simulink model "sampleModel25"  (Simulink 9.1)
settings: Solver=VariableStepAuto  StartTime=0.0  StopTime=10.0  RelTol=1e-3
undefined symbols (not defined in the file): DiscIntNeverNeededParam, Newton, Raphson
libraries: simulink x56
(part 2 of 2)

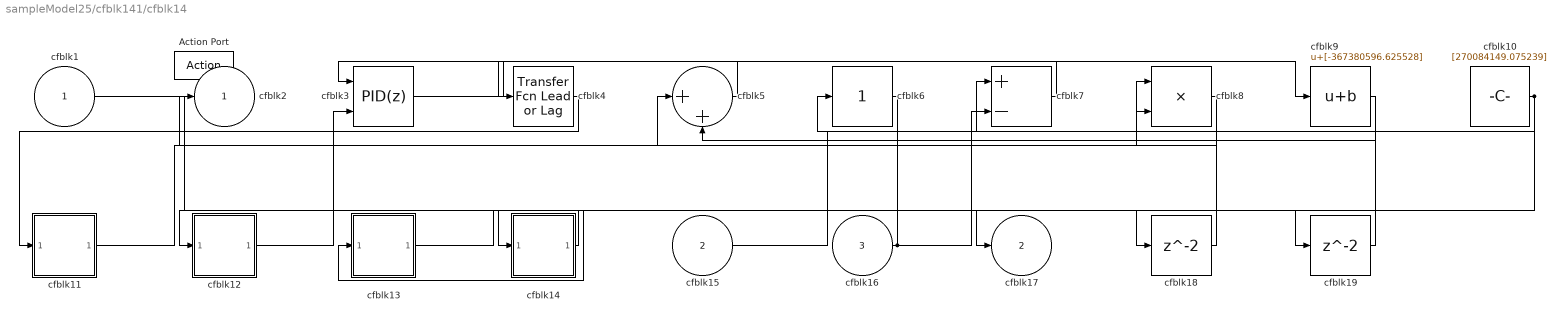
== system sampleModel25/cfblk141/cfblk14 ==
  cfblk1 : Inport
  cfblk15 : Inport  Port=2
  cfblk16 : Inport  Port=3
  Action Port : ActionPort  ActionType=then
  cfblk10 : Constant  Value=[270084149.075239]  SampleTime=1
  cfblk11 : Subsystem
  cfblk12 : Subsystem
  cfblk13 : Subsystem
  cfblk14 : Subsystem
  cfblk18 : Delay
  cfblk19 : Delay
  cfblk3 : simulink/Continuous/PID Controller (2DOF)  Controller=PID  TimeDomain=Discrete-time  SampleTime=-1  IntegratorMethod=Forward Euler  FilterMethod=Forward Euler  Form=Parallel  UseFilter=on  ControllerParametersSource=internal  P=1  I=1  D=0  N=100  b=1  c=1  InitialConditionSource=internal  InitialConditionForIntegrator=0  InitialConditionForFilter=0  ExternalReset=none  LimitOutput=off  UpperSaturationLimit=inf  LowerSaturationLimit=-inf  LinearizeAsGain=off  AntiWindupMode=none  Kb=1  TrackingMode=off  Kt=1  PParamMin=[]  PParamMax=[]  IParamMin=[]  IParamMax=[]  DParamMin=[]  DParamMax=[]  NParamMin=[]  NParamMax=[]  bParamMin=[]  bParamMax=[]  cParamMin=[]  cParamMax=[]  KbParamMin=[]  KbParamMax=[]  KtParamMin=[]  KtParamMax=[]  POutMin=[]  POutMax=[]  IOutMin=[]  IOutMax=[]  DOutMin=[]  DOutMax=[]  NOutMin=[]  NOutMax=[]  bOutMin=[]  bOutMax=[]  cOutMin=[]  cOutMax=[]  KbOutMin=[]  KbOutMax=[]  KtOutMin=[]  KtOutMax=[]  IntegratorOutMin=[]  IntegratorOutMax=[]  FilterOutMin=[]  FilterOutMax=[]  SumOutMin=[]  SumOutMax=[]  Sum1OutMin=[]  Sum1OutMax=[]  Sum2OutMin=[]  Sum2OutMax=[]  Sum3OutMin=[]  Sum3OutMax=[]  SumI1OutMin=[]  SumI1OutMax=[]  SumI2OutMin=[]  SumI2OutMax=[]  SumI3OutMin=[]  SumI3OutMax=[]  SumDOutMin=[]  SumDOutMax=[]  SaturationOutMin=[]  SaturationOutMax=[]  IntegratorContinuousStateAttributes=''  IntegratorStateMustResolveToSignalObject=off  IntegratorRTWStateStorageClass=Auto  FilterContinuousStateAttributes=''  FilterStateMustResolveToSignalObject=off  FilterRTWStateStorageClass=Auto  DifferentiatorICPrevScaledInput=0  DifferentiatorOutMin=[]  DifferentiatorOutMax=[]  FilterDiffOutCoefMin=[]  FilterDiffOutCoefMax=[]  SumDenOutMin=[]  SumDenOutMax=[]  SumNumOutMin=[]  SumNumOutMax=[]  ReciprocalOutMin=[]  ReciprocalOutMax=[]  DivideOutMin=[]  DivideOutMax=[]  TunerSelectOption=Transfer Function Based (PID Tuner App)
  cfblk4 : simulink/Discrete/Transfer Fcn Lead or Lag  PoleZ=0.95  ZeroZ=0.75  ICPrevOutput=0.0  ICPrevInput=0.0  DoSatur=off
      settings: SourceProductName=Simulink  SourceProductBaseCode=SL
  cfblk5 : Sum  Inputs=|++
  cfblk6 : simulink/Math Operations/Slider Gain  gain=1  low=0  high=2
  cfblk7 : Sum  Inputs=+-
  cfblk8 : Product  Inputs=**
  cfblk9 : Bias  Bias=[-367380596.625528]
  cfblk2 : Outport
  cfblk17 : Outport  Port=2
  wires:
  cfblk3/1 -> cfblk9/1
  cfblk4/1 -> cfblk11/1(cfblk1)
  cfblk1/1 -> cfblk14/1(cfblk1)
  cfblk5/1 -> cfblk4/1
  cfblk6/1 -> cfblk13/1(cfblk1)
  cfblk7/1 -> cfblk3/1
  cfblk14/1(cfblk2) -> cfblk12/1(cfblk1)
  cfblk12/1(cfblk2) -> cfblk3/2
  cfblk10/1 -> cfblk17/1, cfblk8/2
  cfblk9/1 -> cfblk5/2
  cfblk11/1(cfblk2) -> cfblk8/1
  cfblk15/1 -> cfblk7/1
  cfblk16/1 -> cfblk7/2, cfblk2/1
  cfblk8/1 -> cfblk18/1
  cfblk18/1 -> cfblk5/1
  cfblk13/1(cfblk2) -> cfblk19/1
  cfblk19/1 -> cfblk6/1

== system sampleModel25/cfblk141/cfblk15 ==
  cfblk1 : Inport
  cfblk12 : Inport  Port=2
  cfblk13 : Inport  Port=3
  cfblk14 : Inport  Port=4
  Action Port : ActionPort  ActionType=else
  cfblk10 : Subsystem
  cfblk11 : Subsystem
  cfblk3 : DiscreteFir
  cfblk4 : simulink/Discrete/Tapped Delay  vinit=0.0  samptime=-1  NumDelays=1  DelayOrder=Oldest  includeCurrent=off
  cfblk5 : simulink/Continuous/PID Controller (2DOF)  Controller=PID  TimeDomain=Discrete-time  SampleTime=-1  IntegratorMethod=Forward Euler  FilterMethod=Forward Euler  Form=Parallel  UseFilter=on  ControllerParametersSource=internal  P=1  I=1  D=0  N=100  b=1  c=1  InitialConditionSource=internal  InitialConditionForIntegrator=0  InitialConditionForFilter=0  ExternalReset=none  LimitOutput=off  UpperSaturationLimit=inf  LowerSaturationLimit=-inf  LinearizeAsGain=off  AntiWindupMode=none  Kb=1  TrackingMode=off  Kt=1  PParamMin=[]  PParamMax=[]  IParamMin=[]  IParamMax=[]  DParamMin=[]  DParamMax=[]  NParamMin=[]  NParamMax=[]  bParamMin=[]  bParamMax=[]  cParamMin=[]  cParamMax=[]  KbParamMin=[]  KbParamMax=[]  KtParamMin=[]  KtParamMax=[]  POutMin=[]  POutMax=[]  IOutMin=[]  IOutMax=[]  DOutMin=[]  DOutMax=[]  NOutMin=[]  NOutMax=[]  bOutMin=[]  bOutMax=[]  cOutMin=[]  cOutMax=[]  KbOutMin=[]  KbOutMax=[]  KtOutMin=[]  KtOutMax=[]  IntegratorOutMin=[]  IntegratorOutMax=[]  FilterOutMin=[]  FilterOutMax=[]  SumOutMin=[]  SumOutMax=[]  Sum1OutMin=[]  Sum1OutMax=[]  Sum2OutMin=[]  Sum2OutMax=[]  Sum3OutMin=[]  Sum3OutMax=[]  SumI1OutMin=[]  SumI1OutMax=[]  SumI2OutMin=[]  SumI2OutMax=[]  SumI3OutMin=[]  SumI3OutMax=[]  SumDOutMin=[]  SumDOutMax=[]  SaturationOutMin=[]  SaturationOutMax=[]  IntegratorContinuousStateAttributes=''  IntegratorStateMustResolveToSignalObject=off  IntegratorRTWStateStorageClass=Auto  FilterContinuousStateAttributes=''  FilterStateMustResolveToSignalObject=off  FilterRTWStateStorageClass=Auto  DifferentiatorICPrevScaledInput=0  DifferentiatorOutMin=[]  DifferentiatorOutMax=[]  FilterDiffOutCoefMin=[]  FilterDiffOutCoefMax=[]  SumDenOutMin=[]  SumDenOutMax=[]  SumNumOutMin=[]  SumNumOutMax=[]  ReciprocalOutMin=[]  ReciprocalOutMax=[]  DivideOutMin=[]  DivideOutMax=[]  TunerSelectOption=Transfer Function Based (PID Tuner App)
  cfblk6 : Abs
  cfblk7 : ComplexToMagnitudeAngle
  cfblk8 : Constant  Value=[-68296175.409686]  SampleTime=1
  cfblk9 : Subsystem
  cfblk2 : Outport
  cfblk15 : Outport  Port=2
  wires:
  cfblk6/1 -> cfblk5/1
  cfblk9/1(cfblk2) -> cfblk11/1(cfblk1)
  cfblk10/1(cfblk2) -> cfblk5/2
  cfblk8/1 -> cfblk4/1
  cfblk13/1 -> cfblk7/1
  cfblk5/1 -> cfblk9/1(cfblk1)
  cfblk4/1 -> cfblk3/1
  cfblk14/1 -> cfblk15/1
  cfblk12/1 -> cfblk2/1
  cfblk1/1 -> cfblk6/1
  cfblk3/1 -> cfblk10/1(cfblk1)

== system sampleModel25/cfblk141/cfblk6 ==
  cfblk1 : Inport
  cfblk2 : Outport
  wires:
  cfblk1/1 -> cfblk2/1

== system sampleModel25/cfblk141/cfblk7 ==
  cfblk1 : Inport
  cfblk2 : Outport
  wires:
  cfblk1/1 -> cfblk2/1

== system sampleModel25/cfblk142/cfblk8 ==
  cfblk1 : Inport
  cfblk2 : Outport
  wires:
  cfblk1/1 -> cfblk2/1

== system sampleModel25/cfblk143/cfblk10 ==
  cfblk1 : Inport
  cfblk2 : Outport
  wires:
  cfblk1/1 -> cfblk2/1

== system sampleModel25/cfblk143/cfblk11 ==
  cfblk1 : Inport
  cfblk2 : Outport
  wires:
  cfblk1/1 -> cfblk2/1

== system sampleModel25/cfblk143/cfblk12 ==
  cfblk1 : Inport
  cfblk2 : Outport
  wires:
  cfblk1/1 -> cfblk2/1

== system sampleModel25/cfblk143/cfblk9 ==
  cfblk1 : Inport
  cfblk2 : Outport
  wires:
  cfblk1/1 -> cfblk2/1

== system sampleModel25/cfblk144/cfblk11 ==
  cfblk1 : Inport
  cfblk2 : Outport
  wires:
  cfblk1/1 -> cfblk2/1

== system sampleModel25/cfblk144/cfblk12 ==
  cfblk1 : Inport
  cfblk2 : Outport
  wires:
  cfblk1/1 -> cfblk2/1

== system sampleModel25/cfblk144/cfblk13 ==
  cfblk1 : Inport
  cfblk2 : Outport
  wires:
  cfblk1/1 -> cfblk2/1

== system sampleModel25/cfblk144/cfblk14 ==
  cfblk1 : Inport
  cfblk2 : Outport
  wires:
  cfblk1/1 -> cfblk2/1

== system sampleModel25/cfblk144/cfblk18 ==
  cfblk1 : Inport
  Action Port : ActionPort  ActionType=then
  cfblk3 : MinMax  Function=max  Inputs=2
  cfblk4 : Subsystem
  cfblk5 : Subsystem
  cfblk6 : Subsystem
  cfblk7 : Subsystem
  cfblk8 : Subsystem
  cfblk9 : Delay
  cfblk2 : Outport
  wires:
  cfblk8/1(cfblk2) -> cfblk4/1(cfblk1), cfblk7/1(cfblk1)
  cfblk6/1(cfblk2) -> cfblk8/1(cfblk1)
  cfblk1/1 -> cfblk3/1
  cfblk4/1(cfblk2) -> cfblk2/1
  cfblk3/1 -> cfblk5/1(cfblk1)
  cfblk5/1(cfblk2) -> cfblk6/1(cfblk1)
  cfblk7/1(cfblk2) -> cfblk9/1
  cfblk9/1 -> cfblk3/2

== system sampleModel25/cfblk144/cfblk19 ==
  cfblk1 : Inport
  cfblk7 : Inport  Port=2
  cfblk8 : Inport  Port=3
  Action Port : ActionPort  ActionType=else
  cfblk3 : simulink/Discrete/Transfer Fcn Lead or Lag  PoleZ=0.95  ZeroZ=0.75  ICPrevOutput=0.0  ICPrevInput=0.0  DoSatur=off
      settings: SourceProductName=Simulink  SourceProductBaseCode=SL
  cfblk4 : ComplexToRealImag
  cfblk5 : DotProduct  InputSameDT=on  OutDataTypeStr=Inherit: Inherit via internal rule
  cfblk6 : Subsystem
  cfblk2 : Outport
  wires:
  cfblk1/1 -> cfblk4/1
  cfblk3/1 -> cfblk2/1
  cfblk8/1 -> cfblk3/1
  cfblk7/1 -> cfblk5/1
  cfblk4/1 -> cfblk5/2
  cfblk4/2 -> cfblk6/1(cfblk1)

== system sampleModel25/cfblk145/cfblk10 ==
  cfblk1 : Inport
  cfblk2 : Outport
  wires:
  cfblk1/1 -> cfblk2/1

== system sampleModel25/cfblk145/cfblk7 ==
  cfblk1 : Inport
  cfblk2 : Outport
  wires:
  cfblk1/1 -> cfblk2/1

== system sampleModel25/cfblk145/cfblk8 ==
  cfblk1 : Inport
  cfblk2 : Outport
  wires:
  cfblk1/1 -> cfblk2/1

== system sampleModel25/cfblk145/cfblk9 ==
  cfblk1 : Inport
  cfblk2 : Outport
  wires:
  cfblk1/1 -> cfblk2/1

== system sampleModel25/cfblk146/cfblk9 ==
  cfblk1 : Inport
  cfblk2 : Outport
  wires:
  cfblk1/1 -> cfblk2/1

== system sampleModel25/cfblk147/cfblk10 ==
  cfblk1 : Inport
  cfblk2 : Outport
  wires:
  cfblk1/1 -> cfblk2/1

== system sampleModel25/cfblk147/cfblk18 ==
  cfblk1 : Inport
  cfblk6 : Inport  Port=2
  cfblk7 : Inport  Port=3
  cfblk8 : Inport  Port=4
  cfblk9 : Inport  Port=5
  Action Port : ActionPort  ActionType=then
  cfblk3 : Product  Inputs=**
  cfblk4 : Subsystem
  cfblk5 : Subsystem
  cfblk2 : Outport
  cfblk10 : Outport  Port=2
  cfblk11 : Outport  Port=3
  wires:
  cfblk7/1 -> cfblk3/1
  cfblk4/1(cfblk2) -> cfblk2/1
  cfblk3/1 -> cfblk10/1
  cfblk8/1 -> cfblk3/2
  cfblk9/1 -> cfblk5/1(cfblk1)
  cfblk5/1(cfblk2) -> cfblk4/1(cfblk1)
  cfblk6/1 -> cfblk11/1

== system sampleModel25/cfblk147/cfblk19 ==
  cfblk1 : Inport
  Action Port : ActionPort  ActionType=else
  cfblk10 : Subsystem
  cfblk11 : Subsystem
  cfblk12 : Subsystem
  cfblk3 : DiscreteFilter
  cfblk4 : DiscreteTransferFcn
  cfblk5 : Sum  Inputs=+
  cfblk6 : Sum  Inputs=|++
  cfblk7 : Subsystem
  cfblk8 : Subsystem
  cfblk9 : Subsystem
  cfblk2 : Outport
  cfblk13 : Outport  Port=2
  wires:
  cfblk8/1(cfblk2) -> cfblk10/1(cfblk1)
  cfblk1/1 -> cfblk3/1
  cfblk10/1(cfblk2) -> cfblk13/1
  cfblk5/1 -> cfblk8/1(cfblk1)
  cfblk6/1 -> cfblk7/1(cfblk1)
  cfblk7/1(cfblk2) -> cfblk9/1(cfblk1)
  cfblk3/1 -> cfblk4/1
  cfblk9/1(cfblk2) -> cfblk11/1(cfblk1)
  cfblk4/1 -> cfblk6/1, cfblk6/2
  cfblk11/1(cfblk2) -> cfblk5/1, cfblk12/1(cfblk1)
  cfblk12/1(cfblk2) -> cfblk2/1

== system sampleModel25/cfblk148/cfblk7 ==
  cfblk1 : Inport
  cfblk2 : Outport
  wires:
  cfblk1/1 -> cfblk2/1

== system sampleModel25/cfblk149/cfblk10 ==
  cfblk1 : Inport
  cfblk2 : Outport
  wires:
  cfblk1/1 -> cfblk2/1

== system sampleModel25/cfblk149/cfblk11 ==
  cfblk1 : Inport
  cfblk2 : Outport
  wires:
  cfblk1/1 -> cfblk2/1

== system sampleModel25/cfblk149/cfblk8 ==
  cfblk1 : Inport
  cfblk2 : Outport
  wires:
  cfblk1/1 -> cfblk2/1

== system sampleModel25/cfblk149/cfblk9 ==
  cfblk1 : Inport
  cfblk2 : Outport
  wires:
  cfblk1/1 -> cfblk2/1

== system sampleModel25/cfblk140/cfblk13/cfblk10 ==
  cfblk1 : Inport
  cfblk2 : Outport
  wires:
  cfblk1/1 -> cfblk2/1

== system sampleModel25/cfblk140/cfblk13/cfblk11 ==
  cfblk1 : Inport
  cfblk2 : Outport
  wires:
  cfblk1/1 -> cfblk2/1

== system sampleModel25/cfblk140/cfblk13/cfblk12 ==
  cfblk1 : Inport
  cfblk2 : Outport
  wires:
  cfblk1/1 -> cfblk2/1

== system sampleModel25/cfblk140/cfblk13/cfblk13 ==
  cfblk1 : Inport
  cfblk2 : Outport
  wires:
  cfblk1/1 -> cfblk2/1

== system sampleModel25/cfblk140/cfblk13/cfblk9 ==
  cfblk1 : Inport
  cfblk2 : Outport
  wires:
  cfblk1/1 -> cfblk2/1

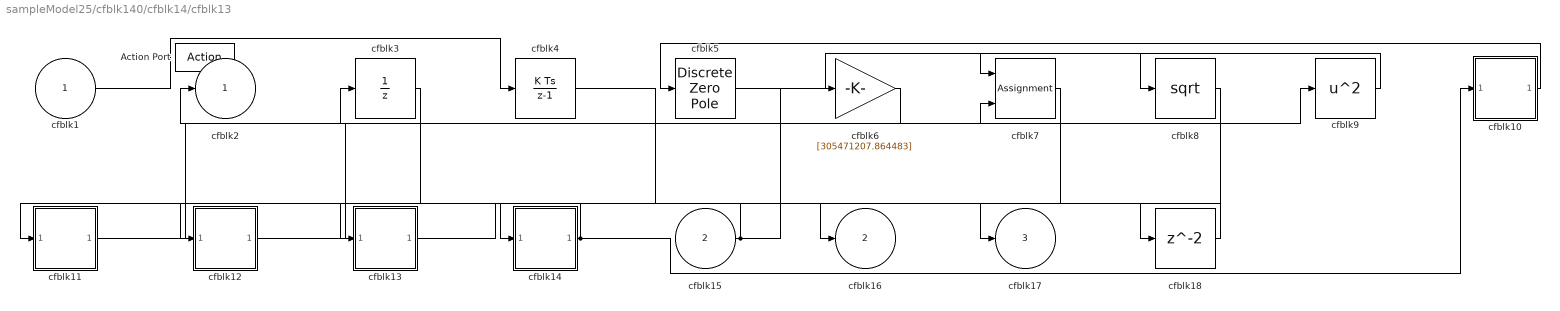
== system sampleModel25/cfblk140/cfblk14/cfblk13 ==
  cfblk1 : Inport
  cfblk15 : Inport  Port=2
  Action Port : ActionPort  ActionType=then
  cfblk10 : Subsystem
  cfblk11 : Subsystem
  cfblk12 : Subsystem
  cfblk13 : Subsystem
  cfblk14 : Subsystem
  cfblk18 : Delay
  cfblk3 : UnitDelay  SampleTime=-1
  cfblk4 : DiscreteIntegrator  SampleTime=-1  ICPrevOutput=DiscIntNeverNeededParam  ICPrevScaledInput=DiscIntNeverNeededParam
  cfblk5 : DiscreteZeroPole  Poles=[0 0.5]  Gain=1  SampleTime=-1
  cfblk6 : Gain  Gain=[305471207.864483]
  cfblk7 : Assignment  DiagnosticForDimensions=Warning  IndexOptions=Index vector (dialog)  Indices=1  OutputSizes=1
  cfblk8 : Sqrt  SaturateOnIntegerOverflow=on
  cfblk9 : Math  Operator=square  SaturateOnIntegerOverflow=on
  cfblk2 : Outport
  cfblk16 : Outport  Port=2
  cfblk17 : Outport  Port=3
  wires:
  cfblk5/1 -> cfblk8/1
  cfblk12/1(cfblk2) -> cfblk9/1
  cfblk1/1 -> cfblk4/1
  cfblk6/1 -> cfblk2/1
  cfblk15/1 -> cfblk14/1(cfblk1), cfblk6/1
  cfblk9/1 -> cfblk7/1
  cfblk14/1(cfblk2) -> cfblk10/1(cfblk1), cfblk11/1(cfblk1)
  cfblk7/1 -> cfblk13/1(cfblk1)
  cfblk8/1 -> cfblk16/1
  cfblk11/1(cfblk2) -> cfblk3/1
  cfblk10/1(cfblk2) -> cfblk5/1
  cfblk4/1 -> cfblk17/1
  cfblk3/1 -> cfblk12/1(cfblk1)
  cfblk13/1(cfblk2) -> cfblk18/1
  cfblk18/1 -> cfblk7/2

== system sampleModel25/cfblk140/cfblk14/cfblk14 ==
  cfblk1 : Inport
  cfblk11 : Inport  Port=2
  Action Port : ActionPort  ActionType=else
  cfblk10 : Subsystem
  cfblk3 : simulink/Discrete/Transfer Fcn Lead or Lag  PoleZ=0.95  ZeroZ=0.75  ICPrevOutput=0.0  ICPrevInput=0.0  DoSatur=off
      settings: SourceProductName=Simulink  SourceProductBaseCode=SL
  cfblk4 : Sin  TimeSource=Use external signal  SampleTime=0
  cfblk5 : Constant  Value=[13372239.767599]  SampleTime=1
  cfblk6 : Constant  Value=[-888197703.177036]  SampleTime=1
  cfblk7 : Subsystem
  cfblk8 : Subsystem
  cfblk9 : Subsystem
  cfblk2 : Outport
  cfblk12 : Outport  Port=2
  wires:
  cfblk1/1 -> cfblk4/1
  cfblk8/1(cfblk2) -> cfblk12/1
  cfblk4/1 -> cfblk8/1(cfblk1)
  cfblk9/1(cfblk2) -> cfblk7/1(cfblk1)
  cfblk5/1 -> cfblk3/1
  cfblk6/1 -> cfblk9/1(cfblk1)
  cfblk3/1 -> cfblk2/1
  cfblk7/1(cfblk2) -> cfblk10/1(cfblk1)

== system sampleModel25/cfblk140/cfblk14/cfblk6 ==
  cfblk1 : Inport
  cfblk2 : Outport
  wires:
  cfblk1/1 -> cfblk2/1

== system sampleModel25/cfblk140/cfblk14/cfblk7 ==
  cfblk1 : Inport
  cfblk2 : Outport
  wires:
  cfblk1/1 -> cfblk2/1

== system sampleModel25/cfblk140/cfblk14/cfblk8 ==
  cfblk1 : Inport
  cfblk2 : Outport
  wires:
  cfblk1/1 -> cfblk2/1

== system sampleModel25/cfblk140/cfblk15/cfblk9 ==
  cfblk1 : Inport
  cfblk2 : Outport
  wires:
  cfblk1/1 -> cfblk2/1

== system sampleModel25/cfblk140/cfblk16/cfblk6 ==
  cfblk1 : Inport
  cfblk2 : Outport
  wires:
  cfblk1/1 -> cfblk2/1

== system sampleModel25/cfblk140/cfblk16/cfblk7 ==
  cfblk1 : Inport
  cfblk2 : Outport
  wires:
  cfblk1/1 -> cfblk2/1

== system sampleModel25/cfblk141/cfblk12/cfblk10 ==
  cfblk1 : Inport
  cfblk2 : Outport
  wires:
  cfblk1/1 -> cfblk2/1

== system sampleModel25/cfblk141/cfblk12/cfblk11 ==
  cfblk1 : Inport
  cfblk2 : Outport
  wires:
  cfblk1/1 -> cfblk2/1

== system sampleModel25/cfblk141/cfblk12/cfblk16 ==
  cfblk1 : Inport
  Action Port : ActionPort  ActionType=then
  cfblk3 : Sqrt  SaturateOnIntegerOverflow=on
  cfblk4 : simulink/Math Operations/MinMax Running Resettable  Function=min  vinit=0.0
  cfblk5 : Constant  Value=[222304569.355251]  SampleTime=1
  cfblk6 : Constant  Value=[-506290689.066987]  SampleTime=1
  cfblk7 : Subsystem
  cfblk8 : Subsystem
  cfblk2 : Outport
  cfblk9 : Outport  Port=2
  wires:
  cfblk6/1 -> cfblk7/1(cfblk1)
  cfblk8/1(cfblk2) -> cfblk9/1
  cfblk5/1 -> cfblk2/1
  cfblk7/1(cfblk2) -> cfblk3/1
  cfblk3/1 -> cfblk4/1
  cfblk4/1 -> cfblk8/1(cfblk1)
  cfblk1/1 -> cfblk4/2

== system sampleModel25/cfblk141/cfblk12/cfblk17 ==
  cfblk1 : Inport
  cfblk13 : Inport  Port=2
  cfblk14 : Inport  Port=3
  cfblk15 : Inport  Port=4
  Action Port : ActionPort  ActionType=else
  cfblk10 : Subsystem
  cfblk11 : Subsystem
  cfblk12 : Subsystem
  cfblk3 : simulink/Discrete/Difference  ICPrevInput=0.0  OutMin=[]  OutMax=[]  OutDataTypeStr=Inherit: Inherit via back propagation  OutDataType=fixdt(1, 16)  OutScaling=2^-10  DoSatur=off
  cfblk4 : simulink/Discrete/Difference  ICPrevInput=0.0  OutMin=[]  OutMax=[]  OutDataTypeStr=Inherit: Inherit via back propagation  OutDataType=fixdt(1, 16)  OutScaling=2^-10  DoSatur=off
  cfblk5 : simulink/Discrete/Transfer Fcn First Order  PoleZ=0.95  ICPrevOutput=0.0  DoSatur=off
      settings: SourceProductName=Simulink
  cfblk6 : Bias  Bias=[920258495.168729]
  cfblk7 : Abs
  cfblk8 : Subsystem
  cfblk9 : Subsystem
  cfblk2 : Outport
  wires:
  cfblk6/1 -> cfblk7/1
  cfblk12/1(cfblk2) -> cfblk2/1
  cfblk1/1 -> cfblk12/1(cfblk1)
  cfblk5/1 -> cfblk4/1
  cfblk8/1(cfblk2) -> cfblk5/1
  cfblk10/1(cfblk2) -> cfblk11/1(cfblk1)
  cfblk11/1(cfblk2) -> cfblk8/1(cfblk1)
  cfblk3/1 -> cfblk6/1
  cfblk9/1(cfblk2) -> cfblk3/1
  cfblk13/1 -> cfblk10/1(cfblk1)
  cfblk15/1 -> cfblk9/1(cfblk1)

== system sampleModel25/cfblk141/cfblk12/cfblk9 ==
  cfblk1 : Inport
  cfblk2 : Outport
  wires:
  cfblk1/1 -> cfblk2/1

== system sampleModel25/cfblk141/cfblk13/cfblk10 ==
  cfblk1 : Inport
  cfblk2 : Outport
  wires:
  cfblk1/1 -> cfblk2/1

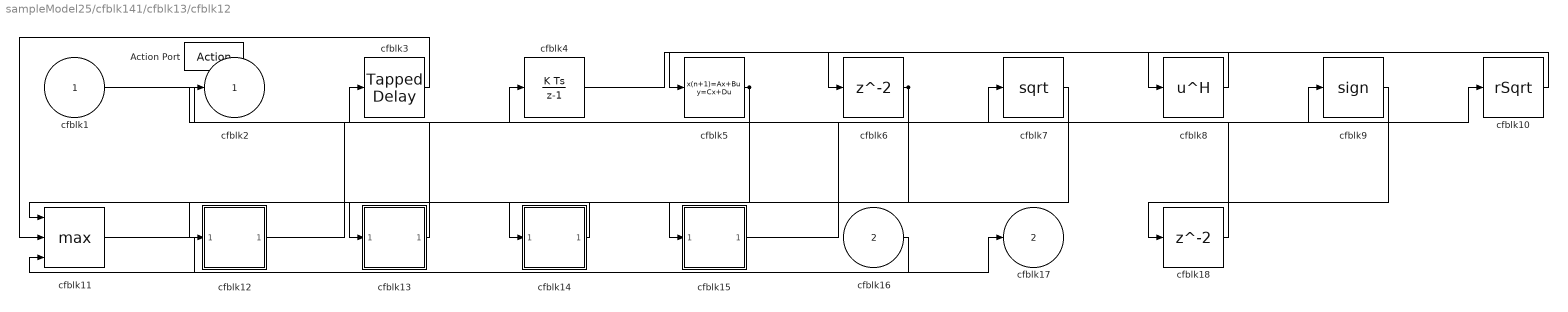
== system sampleModel25/cfblk141/cfblk13/cfblk12 ==
  cfblk1 : Inport
  cfblk16 : Inport  Port=2
  Action Port : ActionPort  ActionType=then
  cfblk10 : Sqrt  Operator=rSqrt  AlgorithmType=Newton-Raphson  SaturateOnIntegerOverflow=on
  cfblk11 : MinMax  Function=max  Inputs=3
  cfblk12 : Subsystem
  cfblk13 : Subsystem
  cfblk14 : Subsystem
  cfblk15 : Subsystem
  cfblk18 : Delay
  cfblk3 : simulink/Discrete/Tapped Delay  vinit=0.0  samptime=-1  NumDelays=1  DelayOrder=Oldest  includeCurrent=off
  cfblk4 : DiscreteIntegrator  SampleTime=-1  ICPrevOutput=DiscIntNeverNeededParam  ICPrevScaledInput=DiscIntNeverNeededParam
  cfblk5 : DiscreteStateSpace  SampleTime=-1
  cfblk6 : Delay
  cfblk7 : Sqrt  SaturateOnIntegerOverflow=on
  cfblk8 : Math  Operator=hermitian  SaturateOnIntegerOverflow=on
  cfblk9 : Signum
  cfblk2 : Outport
  cfblk17 : Outport  Port=2
  wires:
  cfblk6/1 -> cfblk13/1(cfblk1), cfblk15/1(cfblk1)
  cfblk10/1 -> cfblk5/1
  cfblk11/1 -> cfblk17/1
  cfblk15/1(cfblk2) -> cfblk10/1
  cfblk4/1 -> cfblk8/1
  cfblk14/1(cfblk2) -> cfblk12/1(cfblk1)
  cfblk12/1(cfblk2) -> cfblk9/1
  cfblk1/1 -> cfblk7/1
  cfblk8/1 -> cfblk6/1
  cfblk7/1 -> cfblk11/1
  cfblk13/1(cfblk2) -> cfblk3/1
  cfblk3/1 -> cfblk11/2
  cfblk5/1 -> cfblk2/1, cfblk14/1(cfblk1)
  cfblk16/1 -> cfblk11/3
  cfblk9/1 -> cfblk18/1
  cfblk18/1 -> cfblk4/1

== system sampleModel25/cfblk141/cfblk13/cfblk13 ==
  cfblk1 : Inport
  cfblk8 : Inport  Port=2
  cfblk9 : Inport  Port=3
  cfblk10 : Inport  Port=4
  cfblk11 : Inport  Port=5
  Action Port : ActionPort  ActionType=else
  cfblk3 : simulink/Discrete/Difference  ICPrevInput=0.0  OutMin=[]  OutMax=[]  OutDataTypeStr=Inherit: Inherit via back propagation  OutDataType=fixdt(1, 16)  OutScaling=2^-10  DoSatur=off
  cfblk4 : simulink/Continuous/PID Controller  Controller=PID  TimeDomain=Discrete-time  SampleTime=-1  IntegratorMethod=Forward Euler  FilterMethod=Forward Euler  Form=Parallel  UseFilter=on  ControllerParametersSource=internal  P=1  I=1  D=0  N=100  InitialConditionSource=internal  InitialConditionForIntegrator=0  InitialConditionForFilter=0  ExternalReset=none  LimitOutput=off  UpperSaturationLimit=inf  LowerSaturationLimit=-inf  LinearizeAsGain=off  AntiWindupMode=none  Kb=1  TrackingMode=off  Kt=1  PParamMin=[]  PParamMax=[]  IParamMin=[]  IParamMax=[]  DParamMin=[]  DParamMax=[]  NParamMin=[]  NParamMax=[]  KbParamMin=[]  KbParamMax=[]  KtParamMin=[]  KtParamMax=[]  POutMin=[]  POutMax=[]  IOutMin=[]  IOutMax=[]  DOutMin=[]  DOutMax=[]  NOutMin=[]  NOutMax=[]  KbOutMin=[]  KbOutMax=[]  KtOutMin=[]  KtOutMax=[]  IntegratorOutMin=[]  IntegratorOutMax=[]  FilterOutMin=[]  FilterOutMax=[]  SumOutMin=[]  SumOutMax=[]  SumI1OutMin=[]  SumI1OutMax=[]  SumI2OutMin=[]  SumI2OutMax=[]  SumI3OutMin=[]  SumI3OutMax=[]  SumDOutMin=[]  SumDOutMax=[]  SaturationOutMin=[]  SaturationOutMax=[]  IntegratorContinuousStateAttributes=''  IntegratorStateMustResolveToSignalObject=off  IntegratorRTWStateStorageClass=Auto  FilterContinuousStateAttributes=''  FilterStateMustResolveToSignalObject=off  FilterRTWStateStorageClass=Auto  DifferentiatorICPrevScaledInput=0  DifferentiatorOutMin=[]  DifferentiatorOutMax=[]  FilterDiffOutCoefMin=[]  FilterDiffOutCoefMax=[]  SumDenOutMin=[]  SumDenOutMax=[]  SumNumOutMin=[]  SumNumOutMax=[]  ReciprocalOutMin=[]  ReciprocalOutMax=[]  DivideOutMin=[]  DivideOutMax=[]  TunerSelectOption=Transfer Function Based (PID Tuner App)
  cfblk5 : Product  Inputs=**
  cfblk6 : Constant  Value=[-41324313.478639]  SampleTime=1
  cfblk7 : Subsystem
  cfblk2 : Outport
  cfblk12 : Outport  Port=2
  wires:
  cfblk6/1 -> cfblk5/1
  cfblk7/1(cfblk2) -> cfblk2/1
  cfblk5/1 -> cfblk7/1(cfblk1)
  cfblk11/1 -> cfblk5/2
  cfblk1/1 -> cfblk3/1
  cfblk9/1 -> cfblk12/1
  cfblk10/1 -> cfblk4/1

== system sampleModel25/cfblk141/cfblk13/cfblk7 ==
  cfblk1 : Inport
  cfblk2 : Outport
  wires:
  cfblk1/1 -> cfblk2/1

== system sampleModel25/cfblk141/cfblk13/cfblk8 ==
  cfblk1 : Inport
  cfblk2 : Outport
  wires:
  cfblk1/1 -> cfblk2/1

== system sampleModel25/cfblk141/cfblk13/cfblk9 ==
  cfblk1 : Inport
  cfblk2 : Outport
  wires:
  cfblk1/1 -> cfblk2/1

== system sampleModel25/cfblk141/cfblk14/cfblk11 ==
  cfblk1 : Inport
  cfblk2 : Outport
  wires:
  cfblk1/1 -> cfblk2/1

== system sampleModel25/cfblk141/cfblk14/cfblk12 ==
  cfblk1 : Inport
  cfblk2 : Outport
  wires:
  cfblk1/1 -> cfblk2/1

== system sampleModel25/cfblk141/cfblk14/cfblk13 ==
  cfblk1 : Inport
  cfblk2 : Outport
  wires:
  cfblk1/1 -> cfblk2/1

== system sampleModel25/cfblk141/cfblk14/cfblk14 ==
  cfblk1 : Inport
  cfblk2 : Outport
  wires:
  cfblk1/1 -> cfblk2/1

== system sampleModel25/cfblk141/cfblk15/cfblk10 ==
  cfblk1 : Inport
  cfblk2 : Outport
  wires:
  cfblk1/1 -> cfblk2/1

== system sampleModel25/cfblk141/cfblk15/cfblk11 ==
  cfblk1 : Inport
  cfblk2 : Outport
  wires:
  cfblk1/1 -> cfblk2/1

== system sampleModel25/cfblk141/cfblk15/cfblk9 ==
  cfblk1 : Inport
  cfblk2 : Outport
  wires:
  cfblk1/1 -> cfblk2/1

== system sampleModel25/cfblk144/cfblk18/cfblk4 ==
  cfblk1 : Inport
  cfblk2 : Outport
  wires:
  cfblk1/1 -> cfblk2/1

== system sampleModel25/cfblk144/cfblk18/cfblk5 ==
  cfblk1 : Inport
  cfblk2 : Outport
  wires:
  cfblk1/1 -> cfblk2/1

== system sampleModel25/cfblk144/cfblk18/cfblk6 ==
  cfblk1 : Inport
  cfblk2 : Outport
  wires:
  cfblk1/1 -> cfblk2/1

== system sampleModel25/cfblk144/cfblk18/cfblk7 ==
  cfblk1 : Inport
  cfblk2 : Outport
  wires:
  cfblk1/1 -> cfblk2/1

== system sampleModel25/cfblk144/cfblk18/cfblk8 ==
  cfblk1 : Inport
  cfblk2 : Outport
  wires:
  cfblk1/1 -> cfblk2/1

== system sampleModel25/cfblk144/cfblk19/cfblk6 ==
  cfblk1 : Inport
  cfblk2 : Outport
  wires:
  cfblk1/1 -> cfblk2/1

== system sampleModel25/cfblk147/cfblk18/cfblk4 ==
  cfblk1 : Inport
  cfblk2 : Outport
  wires:
  cfblk1/1 -> cfblk2/1

== system sampleModel25/cfblk147/cfblk18/cfblk5 ==
  cfblk1 : Inport
  cfblk2 : Outport
  wires:
  cfblk1/1 -> cfblk2/1

== system sampleModel25/cfblk147/cfblk19/cfblk10 ==
  cfblk1 : Inport
  cfblk2 : Outport
  wires:
  cfblk1/1 -> cfblk2/1

== system sampleModel25/cfblk147/cfblk19/cfblk11 ==
  cfblk1 : Inport
  cfblk2 : Outport
  wires:
  cfblk1/1 -> cfblk2/1

== system sampleModel25/cfblk147/cfblk19/cfblk12 ==
  cfblk1 : Inport
  cfblk2 : Outport
  wires:
  cfblk1/1 -> cfblk2/1

== system sampleModel25/cfblk147/cfblk19/cfblk7 ==
  cfblk1 : Inport
  cfblk2 : Outport
  wires:
  cfblk1/1 -> cfblk2/1

== system sampleModel25/cfblk147/cfblk19/cfblk8 ==
  cfblk1 : Inport
  cfblk2 : Outport
  wires:
  cfblk1/1 -> cfblk2/1

== system sampleModel25/cfblk147/cfblk19/cfblk9 ==
  cfblk1 : Inport
  cfblk2 : Outport
  wires:
  cfblk1/1 -> cfblk2/1

== system sampleModel25/cfblk140/cfblk14/cfblk13/cfblk10 ==
  cfblk1 : Inport
  cfblk2 : Outport
  wires:
  cfblk1/1 -> cfblk2/1

== system sampleModel25/cfblk140/cfblk14/cfblk13/cfblk11 ==
  cfblk1 : Inport
  cfblk2 : Outport
  wires:
  cfblk1/1 -> cfblk2/1

== system sampleModel25/cfblk140/cfblk14/cfblk13/cfblk12 ==
  cfblk1 : Inport
  cfblk2 : Outport
  wires:
  cfblk1/1 -> cfblk2/1

== system sampleModel25/cfblk140/cfblk14/cfblk13/cfblk13 ==
  cfblk1 : Inport
  cfblk2 : Outport
  wires:
  cfblk1/1 -> cfblk2/1

== system sampleModel25/cfblk140/cfblk14/cfblk13/cfblk14 ==
  cfblk1 : Inport
  cfblk2 : Outport
  wires:
  cfblk1/1 -> cfblk2/1

== system sampleModel25/cfblk140/cfblk14/cfblk14/cfblk10 ==
  cfblk1 : Inport
  cfblk2 : Outport
  wires:
  cfblk1/1 -> cfblk2/1

== system sampleModel25/cfblk140/cfblk14/cfblk14/cfblk7 ==
  cfblk1 : Inport
  cfblk2 : Outport
  wires:
  cfblk1/1 -> cfblk2/1

== system sampleModel25/cfblk140/cfblk14/cfblk14/cfblk8 ==
  cfblk1 : Inport
  cfblk2 : Outport
  wires:
  cfblk1/1 -> cfblk2/1

== system sampleModel25/cfblk140/cfblk14/cfblk14/cfblk9 ==
  cfblk1 : Inport
  cfblk2 : Outport
  wires:
  cfblk1/1 -> cfblk2/1

== system sampleModel25/cfblk141/cfblk12/cfblk16/cfblk7 ==
  cfblk1 : Inport
  cfblk2 : Outport
  wires:
  cfblk1/1 -> cfblk2/1

== system sampleModel25/cfblk141/cfblk12/cfblk16/cfblk8 ==
  cfblk1 : Inport
  cfblk2 : Outport
  wires:
  cfblk1/1 -> cfblk2/1

== system sampleModel25/cfblk141/cfblk12/cfblk17/cfblk10 ==
  cfblk1 : Inport
  cfblk2 : Outport
  wires:
  cfblk1/1 -> cfblk2/1

== system sampleModel25/cfblk141/cfblk12/cfblk17/cfblk11 ==
  cfblk1 : Inport
  cfblk2 : Outport
  wires:
  cfblk1/1 -> cfblk2/1

== system sampleModel25/cfblk141/cfblk12/cfblk17/cfblk12 ==
  cfblk1 : Inport
  cfblk2 : Outport
  wires:
  cfblk1/1 -> cfblk2/1

== system sampleModel25/cfblk141/cfblk12/cfblk17/cfblk8 ==
  cfblk1 : Inport
  cfblk2 : Outport
  wires:
  cfblk1/1 -> cfblk2/1

== system sampleModel25/cfblk141/cfblk12/cfblk17/cfblk9 ==
  cfblk1 : Inport
  cfblk2 : Outport
  wires:
  cfblk1/1 -> cfblk2/1

== system sampleModel25/cfblk141/cfblk13/cfblk12/cfblk12 ==
  cfblk1 : Inport
  cfblk2 : Outport
  wires:
  cfblk1/1 -> cfblk2/1

== system sampleModel25/cfblk141/cfblk13/cfblk12/cfblk13 ==
  cfblk1 : Inport
  cfblk2 : Outport
  wires:
  cfblk1/1 -> cfblk2/1

== system sampleModel25/cfblk141/cfblk13/cfblk12/cfblk14 ==
  cfblk1 : Inport
  cfblk2 : Outport
  wires:
  cfblk1/1 -> cfblk2/1

== system sampleModel25/cfblk141/cfblk13/cfblk12/cfblk15 ==
  cfblk1 : Inport
  cfblk2 : Outport
  wires:
  cfblk1/1 -> cfblk2/1

== system sampleModel25/cfblk141/cfblk13/cfblk13/cfblk7 ==
  cfblk1 : Inport
  cfblk2 : Outport
  wires:
  cfblk1/1 -> cfblk2/1
